simulink model "bldcModel_r2017a"  (R2017a)
settings: Solver=VariableStepAuto  StartTime=0.0  StopTime=10.0  RelTol=1e-3
settings Model: Creator=tdarrah  LastModifiedBy=tdarrah

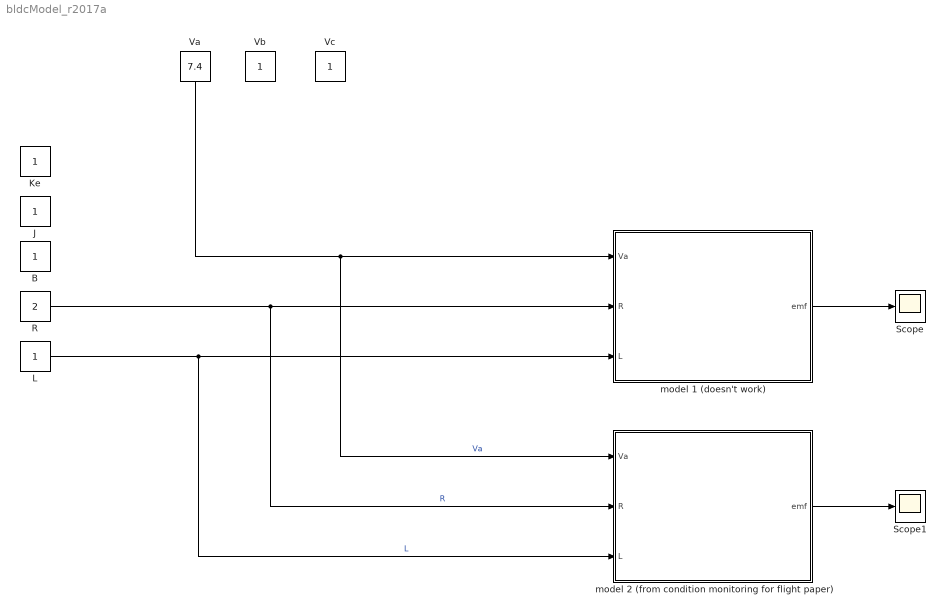
== system bldcModel_r2017a ==
  B : Constant
  J : Constant
  Ke : Constant
  L : Constant
  R : Constant  Value=2
  Scope : Scope
  Scope1 : Scope
  Va : Constant  Value=7.4
  Vb : Constant
  Vc : Constant
  model 1 (doesn't work) : Subsystem
  model 2 (from condition monitoring for flight paper) : Subsystem
  wires:
  Va/1 -> model 2 (from condition monitoring for flight paper)/1(Va), model 1 (doesn't work)/1(Va)  "Va"
  R/1 -> model 2 (from condition monitoring for flight paper)/2(R), model 1 (doesn't work)/2(R)  "R"
  L/1 -> model 2 (from condition monitoring for flight paper)/3(L), model 1 (doesn't work)/3(L)  "L"
  model 1 (doesn't work)/1(emf) -> Scope/1
  model 2 (from condition monitoring for flight paper)/1(emf) -> Scope1/1

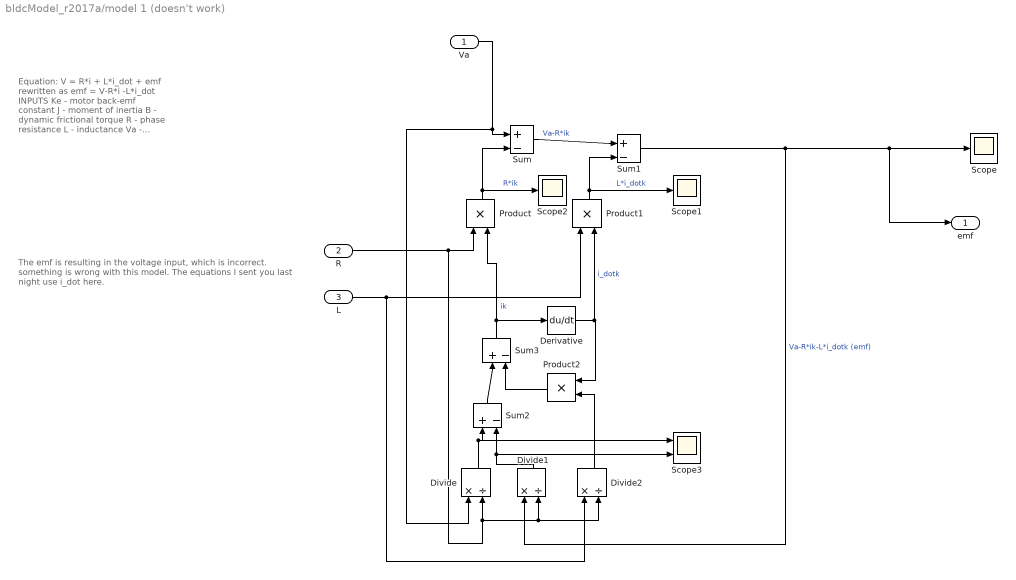
== system bldcModel_r2017a/model 1 (doesn't work) ==
  note: Equation: V = R*i + L*i_dot + emf
      |
      | rewritten as emf = V-R*i -L*i_dot
      |
      | INPUTS
      | Ke - motor back-emf constant
      | J - moment of inertia
      | B - dynamic frictional torque
      | R - phase resistance
      | L - inductance
      | Va - voltage
      | Vb - voltage
      | Vc - voltage
  note: The emf is resulting in the voltage input, which is incorrect.
      | something is wrong with this model. The equations I sent you
      | last night use i_dot here.
  Va : Inport
  R : Inport  Port=2
  L : Inport  Port=3
  Derivative : Derivative
  Divide : Product  Inputs=*/
  Divide1 : Product  Inputs=*/
  Divide2 : Product  Inputs=*/
  Product : Product
  Product1 : Product
  Product2 : Product
  Scope : Scope
  Scope1 : Scope
  Scope2 : Scope
  Scope3 : Scope  NumInputPorts=2
  Sum{,1..3} (4 alike) : Sum  Inputs=+|-
  emf : Outport
  wires:
  R/1 -> Product/1, Divide2/2, Divide1/2, Divide/2
  Va/1 -> Divide/1, Sum/1
  Product/1 -> Scope2/1, Sum/2  "R*ik"
  Sum/1 -> Sum1/1  "Va-R*ik"
  Divide/1 -> Sum2/1, Scope3/1
  Divide1/1 -> Sum2/2, Scope3/2
  L/1 -> Product1/1, Divide2/1
  Sum1/1 -> emf/1, Scope/1, Divide1/1  "Va-R*ik-L*i_dotk (emf)"
  Divide2/1 -> Product2/2
  Sum3/1 -> Product/2, Derivative/1  "ik"
  Sum2/1 -> Sum3/1
  Derivative/1 -> Product2/1, Product1/2  "i_dotk"
  Product2/1 -> Sum3/2
  Product1/1 -> Scope1/1, Sum1/2  "L*i_dotk"

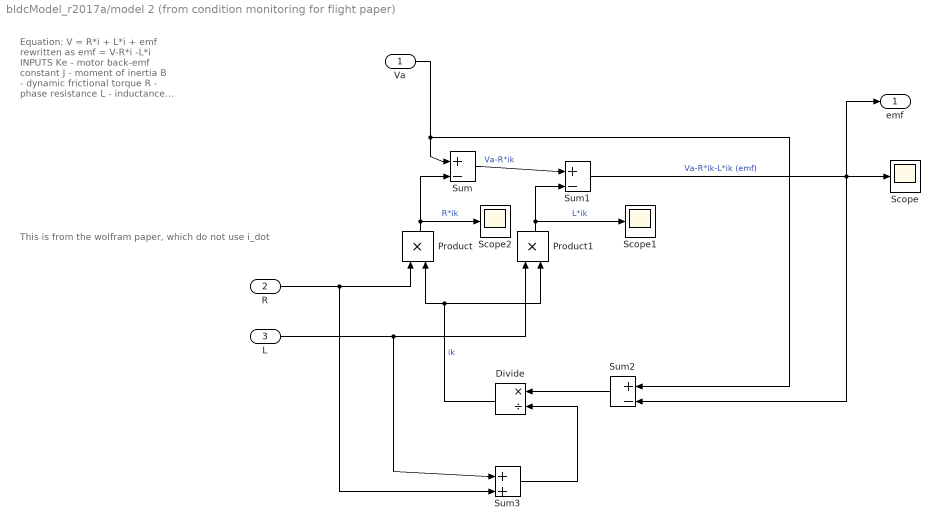
== system bldcModel_r2017a/model 2 (from condition monitoring for flight paper) ==
  note: Equation: V = R*i + L*i + emf
      |
      | rewritten as emf = V-R*i -L*i
      |
      | INPUTS
      | Ke - motor back-emf constant
      | J - moment of inertia
      | B - dynamic frictional torque
      | R - phase resistance
      | L - inductance
      | Va - voltage
      | Vb - voltage
      | Vc - voltage
  note: This is from the wolfram paper, which do not use i_dot
  Va : Inport
  R : Inport  Port=2
  L : Inport  Port=3
  Divide : Product  Inputs=*/
  Product : Product
  Product1 : Product
  Scope : Scope
  Scope1 : Scope
  Scope2 : Scope
  Sum : Sum  Inputs=+|-
  Sum1 : Sum  Inputs=+|-
  Sum2 : Sum  Inputs=+|-
  Sum3 : Sum  Inputs=+|+
  emf : Outport
  wires:
  R/1 -> Sum3/2, Product/1
  Va/1 -> Sum2/1, Sum/1
  Product/1 -> Scope2/1, Sum/2  "R*ik"
  Sum/1 -> Sum1/1  "Va-R*ik"
  L/1 -> Sum3/1, Product1/1
  Sum1/1 -> emf/1, Sum2/2, Scope/1  "Va-R*ik-L*ik (emf)"
  Product1/1 -> Scope1/1, Sum1/2  "L*ik"
  Divide/1 -> Product/2, Product1/2  "ik"
  Sum2/1 -> Divide/1
  Sum3/1 -> Divide/2
